simulink model "wuty_HM"  (R2019a)
settings: Solver=FixedStepAuto  StartTime=0.0  StopTime=10000  FixedStep=1  RelTol=1e-3  EnableMultiTasking=on
libraries: arduinolib x8
settings Model: SnapshotBufferSize=100  SnapshotInterval=1  ExtModeTrigDuration=2  Creator=dell  LastModifiedBy=wuty
settings SolverCC: AutoInsertRateTranBlk=on
settings DataIOCC: LimitDataPoints=on  ReturnWorkspaceOutputs=off
settings OptimizationCC: EnhancedBackFolding=on  PassReuseOutputArgsAs=Individual arguments  ZeroExternalMemoryAtStartup=off  ZeroInternalMemoryAtStartup=off  MaxStackSize=64  OptimizeBlockOrder=speed  DifferentSizesBufferReuse=on  OptimizationCustomize=off
settings DebuggingCC: ParameterTunabilityLossMsg=error  AllowSymbolicDim=off  SFUnexpectedBacktrackingDiag=warning  SFNoUnconditionalDefaultTransitionDiag=warning  SFExecutionAtInitializationDiag=none  ArithmeticOperatorsInVariantConditions=warning
settings HardwareCC: ProdBitPerInt=16  ProdBitPerPointer=16  ProdBitPerSizeT=16  ProdBitPerPtrDiffT=16  ProdLargestAtomicFloat=None  ProdWordSize=8  ProdHWDeviceType=Atmel->AVR  UseEmbeddedCoderFeatures=off
settings SFSimCC: SimUseLocalCustomCode=off  MATLABDynamicMemAlloc=off
settings RTWCC: SystemTargetFile=ert.tlc  HardwareBoard=Arduino Uno  TLCOptions=-aInlineSetEventsForThisBaseRateFcn=TLC_FALSE -aSuppressMultiTaskScheduler=TLC_FALSE -aRateBasedStepFcn=1  TemplateMakefile=ert_default_tmf  GenerateReport=on  RTWUseLocalCustomCode=off  Toolchain=Arduino AVR  BuildConfiguration=Faster Runs  IncludeHyperlinkInReport=on  LaunchReport=on  GenerateTraceInfo=on  GenerateTraceReport=on  GenerateTraceReportSl=on  GenerateTraceReportSf=on  GenerateTraceReportEml=on
settings CodeAppCC: ForceParamTrailComments=on  IgnoreCustomStorageClasses=off  OperatorAnnotations=on  SimulinkDataObjDesc=on  SFDataObjDesc=on  InsertBlockDesc=on
settings ERTTargetCC: SupportContinuousTime=on  SupportNonInlinedSFcns=on  SupportVariableSizeSignals=on  ExtModeStaticAllocSize=250
settings ConfigComp: CovMetricSettings=dw  CovHtmlReporting=on  CovSaveCumulativeToWorkspaceVar=on  CovSaveSingleToWorkspaceVar=on  CovShowResultsExplorer=off  CovExternalEMLEnable=off

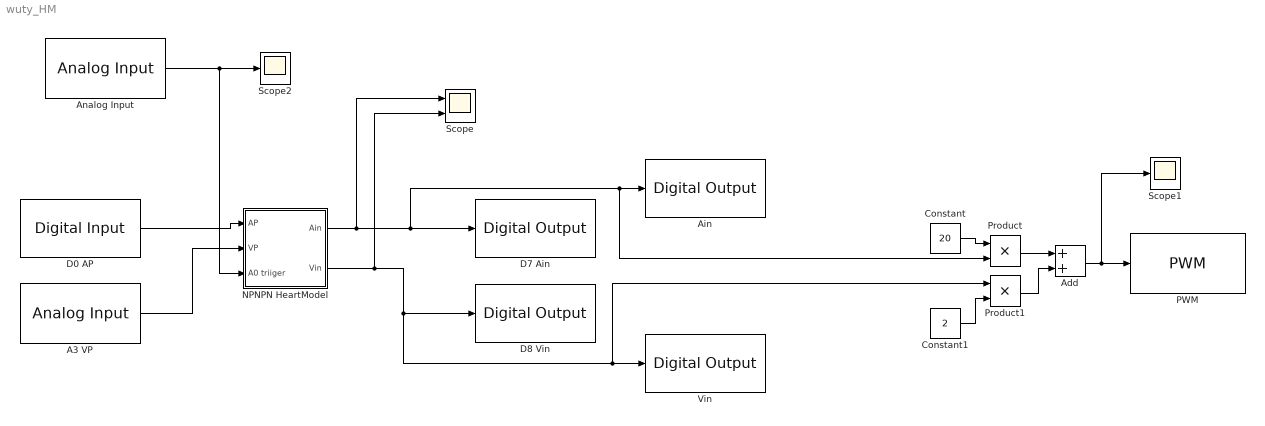
== system wuty_HM ==
  A3 VP : arduinolib/Analog Input  pinNumber=3  ReadResultsOnly=off  ConversionTriggerSource=Software  ExternalTriggerType=uint32(0)  OutputDataType=uint16  EnableConversionCompleteNotify=off  EnableOuputStatus=off  SampleTime=inf  blockPlatform=arduino
  Add : Sum
  Ain : arduinolib/Digital Output  pinNumber=13  blockPlatform=arduino
  Analog Input : arduinolib/Analog Input  pinNumber=0  ReadResultsOnly=off  ConversionTriggerSource=Software  ExternalTriggerType=uint32(0)  OutputDataType=uint16  EnableConversionCompleteNotify=off  EnableOuputStatus=off  SampleTime=inf  blockPlatform=arduino
  Constant : Constant  Value=20
  Constant1 : Constant  Value=2
  D0 AP : arduinolib/Digital Input  pinNumber=0  sampleTime=inf  blockPlatform=arduino
      settings: SourceProductName=Simulink Support Package for Arduino Hardware
  D7 Ain : arduinolib/Digital Output  pinNumber=7  blockPlatform=arduino
  D8 Vin : arduinolib/Digital Output  pinNumber=8  blockPlatform=arduino
  NPNPN HeartModel : Subsystem
  PWM : arduinolib/PWM  pinNumber=5  EnableInputFrequency=off  InitialFrequency=2000  InitialDutyCycle=0  NotificationType=None  blockPlatform=arduino
  Product : Product
  Product1 : Product
  Scope : Scope  NumInputPorts=2
  Scope1 : Scope
  Scope2 : Scope
  Vin : arduinolib/Digital Output  pinNumber=12  blockPlatform=arduino
  wires:
  NPNPN HeartModel/1(Ain) -> Scope/1, Product/2, Ain/1, D7 Ain/1
  NPNPN HeartModel/2(Vin) -> Scope/2, Product1/1, Vin/1, D8 Vin/1
  D0 AP/1 -> NPNPN HeartModel/1(AP)
  A3 VP/1 -> NPNPN HeartModel/2(VP)
  Add/1 -> Scope1/1, PWM/1
  Product/1 -> Add/1
  Constant/1 -> Product/1
  Product1/1 -> Add/2
  Constant1/1 -> Product1/2
  Analog Input/1 -> NPNPN HeartModel/3("A0 triiger "), Scope2/1

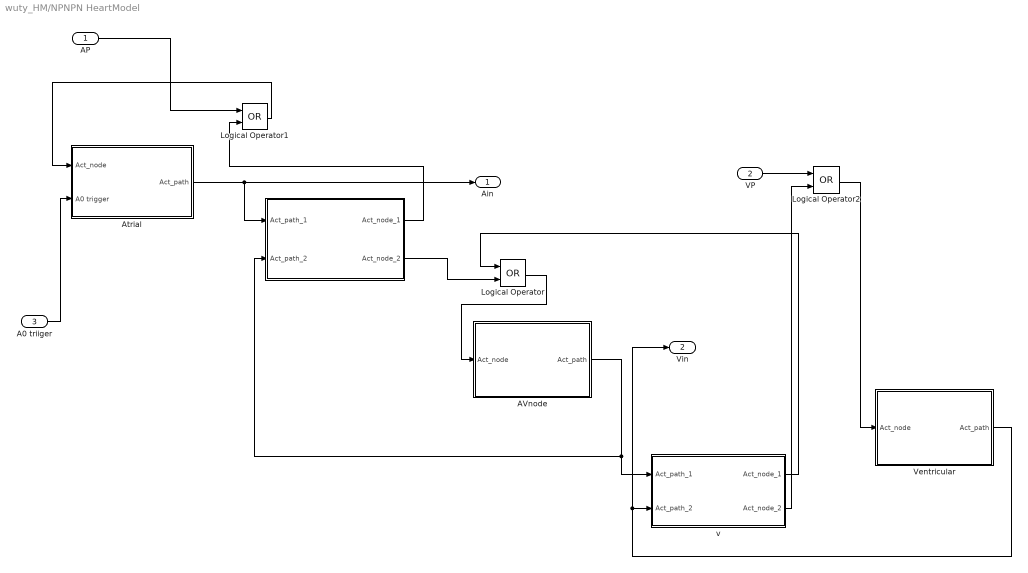
== system wuty_HM/NPNPN HeartModel ==
  AP : Inport
  VP : Inport  Port=2
  "A0 triiger " : Inport  Port=3
  " " : Subsystem  AncestorBlock=model_library/Path
  AVnode : Subsystem  AncestorBlock=model_library/Node
  Atrial : Subsystem  AncestorBlock=model_library/Node
  Logical Operator : Logic  Operator=OR  AllPortsSameDT=off  OutDataTypeStr=boolean
  Logical Operator1 : Logic  Operator=OR  AllPortsSameDT=off  OutDataTypeStr=boolean
  Logical Operator2 : Logic  Operator=OR  AllPortsSameDT=off  OutDataTypeStr=boolean
  Ventricular : Subsystem  AncestorBlock=model_library/Node
  v : Subsystem  AncestorBlock=model_library/Path
  Ain : Outport  VectorParamsAs1DForOutWhenUnconnected=on
  Vin : Outport  Port=2  VectorParamsAs1DForOutWhenUnconnected=on
  wires:
  v/1(Act_node_1) -> Logical Operator/1
  AVnode/1(Act_path) -> " "/2(Act_path_2), v/1(Act_path_1)
  Ventricular/1(Act_path) -> v/2(Act_path_2), Vin/1
  Logical Operator1/1 -> Atrial/1(Act_node)
  Logical Operator/1 -> AVnode/1(Act_node)
  " "/1(Act_node_1) -> Logical Operator1/2
  Logical Operator2/1 -> Ventricular/1(Act_node)
  " "/2(Act_node_2) -> Logical Operator/2
  v/2(Act_node_2) -> Logical Operator2/2
  Atrial/1(Act_path) -> Ain/1, " "/1(Act_path_1)
  "A0 triiger "/1 -> Atrial/2(A0 trigger)
  AP/1 -> Logical Operator1/1
  VP/1 -> Logical Operator2/1

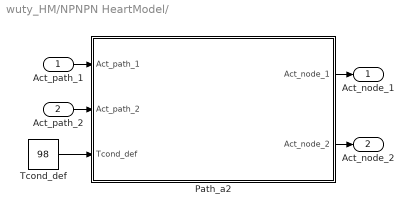
== system wuty_HM/NPNPN HeartModel/  ==
  Act_path_1 : Inport
  Act_path_2 : Inport  Port=2
  Path_a2 : Stateflow chart  TreatAsAtomicUnit=on
  Tcond_def : Constant  Value=98  OutDataTypeStr=uint16
  Act_node_1 : Outport
  Act_node_2 : Outport  Port=2
  wires:
  Tcond_def/1 -> Path_a2/3(Tcond_def)
  Path_a2/2(Act_node_2) -> Act_node_2/1
  Act_path_1/1 -> Path_a2/1(Act_path_1)
  Act_path_2/1 -> Path_a2/2(Act_path_2)
  Path_a2/1(Act_node_1) -> Act_node_1/1

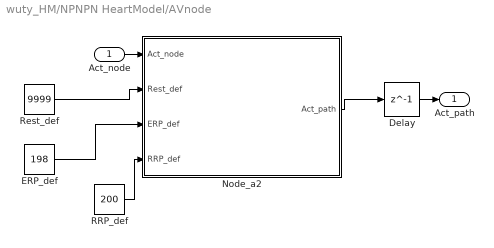
== system wuty_HM/NPNPN HeartModel/AVnode ==
  Act_node : Inport
  Delay : Delay  DelayLength=1  InitialCondition=0
  ERP_def : Constant  Value=198  OutDataTypeStr=uint16
  Node_a2 : Stateflow chart  TreatAsAtomicUnit=on
  RRP_def : Constant  Value=200  OutDataTypeStr=uint16
  Rest_def : Constant  Value=9999  OutDataTypeStr=uint16
  Act_path : Outport
  wires:
  RRP_def/1 -> Node_a2/4(RRP_def)
  Delay/1 -> Act_path/1
  ERP_def/1 -> Node_a2/3(ERP_def)
  Rest_def/1 -> Node_a2/2(Rest_def)
  Act_node/1 -> Node_a2/1(Act_node)
  Node_a2/1(Act_path) -> Delay/1

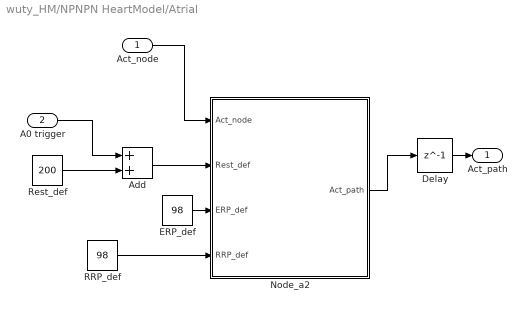
== system wuty_HM/NPNPN HeartModel/Atrial ==
  Act_node : Inport
  A0 trigger : Inport  Port=2
  Add : Sum
  Delay : Delay  DelayLength=1  InitialCondition=0
  ERP_def : Constant  Value=98  OutDataTypeStr=uint16
  Node_a2 : Stateflow chart  TreatAsAtomicUnit=on
  RRP_def : Constant  Value=98  OutDataTypeStr=uint16
  Rest_def : Constant  Value=200  OutDataTypeStr=uint16
  Act_path : Outport
  wires:
  RRP_def/1 -> Node_a2/4(RRP_def)
  Delay/1 -> Act_path/1
  ERP_def/1 -> Node_a2/3(ERP_def)
  Act_node/1 -> Node_a2/1(Act_node)
  Node_a2/1(Act_path) -> Delay/1
  Rest_def/1 -> Add/2
  A0 trigger/1 -> Add/1
  Add/1 -> Node_a2/2(Rest_def)

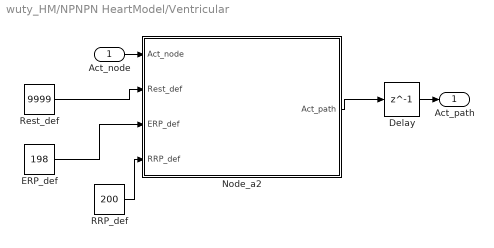
== system wuty_HM/NPNPN HeartModel/Ventricular ==
  Act_node : Inport
  Delay : Delay  DelayLength=1  InitialCondition=0
  ERP_def : Constant  Value=198  OutDataTypeStr=uint16
  Node_a2 : Stateflow chart  TreatAsAtomicUnit=on
  RRP_def : Constant  Value=200  OutDataTypeStr=uint16
  Rest_def : Constant  Value=9999  OutDataTypeStr=uint16
  Act_path : Outport
  wires:
  RRP_def/1 -> Node_a2/4(RRP_def)
  Delay/1 -> Act_path/1
  ERP_def/1 -> Node_a2/3(ERP_def)
  Rest_def/1 -> Node_a2/2(Rest_def)
  Act_node/1 -> Node_a2/1(Act_node)
  Node_a2/1(Act_path) -> Delay/1

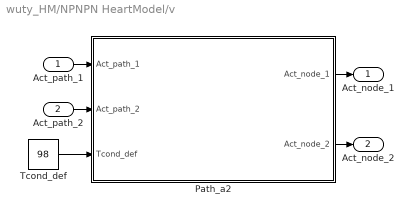
== system wuty_HM/NPNPN HeartModel/v ==
  Act_path_1 : Inport
  Act_path_2 : Inport  Port=2
  Path_a2 : Stateflow chart  TreatAsAtomicUnit=on
  Tcond_def : Constant  Value=98  OutDataTypeStr=uint16
  Act_node_1 : Outport
  Act_node_2 : Outport  Port=2
  wires:
  Tcond_def/1 -> Path_a2/3(Tcond_def)
  Path_a2/2(Act_node_2) -> Act_node_2/1
  Act_path_1/1 -> Path_a2/1(Act_path_1)
  Act_path_2/1 -> Path_a2/2(Act_path_2)
  Path_a2/1(Act_node_1) -> Act_node_1/1

== stateflow chart wuty_HM/NPNPN HeartModel/AVnode/Node_a2 ==
  state node
    settings: description=|
        | temp can be thought of a sub-mode of ERP, which only exists to make sure that act_path is high for one period.
        | 
        | In ERP, if Act_node is received, then it is ignored through that self-transition.
        | 
        | Note this doesn't model variations in cycle length because everytime it is stimulated in RRP, ERP_cur is set to ERP_def again.
    state Rest
    state RRP
    state ERP
    state temp
    (default) -> Rest : {Rest_cur=Rest_def;}
    Rest -> temp [order 3] : [Act_node==false && Rest_cur<=uint16(0)]/{Act_path=true;uptime= uint16(0);ERP_cur=ERP_def;}
    Rest -> temp [order 1] : [Act_node==true]/{Act_path=true;uptime= uint16(0);ERP_cur=ERP_def;}
    Rest -> Rest [order 2] : [Act_node==false && Rest_cur>uint16(0)]/{Rest_cur = Rest_cur - uint16(1);}
    RRP -> Rest [order 1] : [RRP_cur<=0]/{Rest_cur=Rest_def;}
    RRP -> RRP [order 2] : [Act_node==false && RRP_cur>0]/{RRP_cur=RRP_cur-uint16(1);}
    RRP -> temp [order 3] : [Act_node==true]/{Act_path=true;uptime= uint16(0);ERP_cur=ERP_def;}
    ERP -> RRP [order 1] : [ERP_cur<=uint16(0)]/{RRP_cur=RRP_def;}
    temp -> temp [order 1] : [uptime<uint16(1)]/{uptime = uptime + uint16(1);ERP_cur =ERP_cur - uint16(1);}
    temp -> ERP [order 2] : [uptime>=uint16(1)]/{Act_path=false;}
    ERP -> ERP [order 3] : [Act_node==true]
    ERP -> ERP [order 2] : {ERP_cur = ERP_cur - uint16(1);}
  data: Act_node input boolean; Act_path output boolean; Rest_cur local uint16; ERP_cur local uint16; Rest_def input uint16; ERP_def input uint16; uptime local uint16; RRP_cur local uint16; RRP_def input uint16

== stateflow chart wuty_HM/NPNPN HeartModel/v/Path_a2 ==
  state path
    state Idle
    state Ante
    state Retro
    state Wait
    (default) -> Idle
    Idle -> Ante [order 1] : [Act_path_1==true]/{Tcond_cur=Tcond_def;}
    Idle -> Retro [order 2] : [Act_path_2==true]/{Tcond_cur=Tcond_def;}
    Wait -> Idle [order 1] : [uptime>0]/{Act_node_1=false;Act_node_2=false;}
    Ante -> Ante [order 3] : [Act_path_2==false && Tcond_cur>uint16(0)]/{Tcond_cur = Tcond_cur - uint16(1);}
    Retro -> Retro [order 3] : [Act_path_1==false && Tcond_cur>uint16(0)]/{Tcond_cur = Tcond_cur - uint16(1);}
    Ante -> Wait [order 2] : [Act_path_2==true]/{uptime=uint16(0);}
    Ante -> Wait [order 1] : [Act_path_2==false && Tcond_cur<=uint16(0)]/{Act_node_2=true;uptime=uint16(0);}
    Retro -> Wait [order 2] : [Act_path_1==true]/{uptime=uint16(0);}
    Retro -> Wait [order 1] : [Act_path_1==false && Tcond_cur<=uint16(0)]/{Act_node_1=true;uptime=uint16(0);}
    Wait -> Wait [order 2] : [uptime<=uint16(0)]/{uptime = uptime + uint16(1);}
  data: Act_path_1 input boolean; Act_path_2 input boolean; Act_node_1 output boolean; Act_node_2 output boolean; Tcond_cur local uint16; Tcond_def input uint16; uptime local uint16

== stateflow chart wuty_HM/NPNPN HeartModel/Ventricular/Node_a2 ==
  state node
    settings: description=|
        | temp can be thought of a sub-mode of ERP, which only exists to make sure that act_path is high for one period.
        | 
        | In ERP, if Act_node is received, then it is ignored through that self-transition.
        | 
        | Note this doesn't model variations in cycle length because everytime it is stimulated in RRP, ERP_cur is set to ERP_def again.
    state Rest
    state RRP
    state ERP
    state temp
    (default) -> Rest : {Rest_cur=Rest_def;}
    Rest -> temp [order 3] : [Act_node==false && Rest_cur<=uint16(0)]/{Act_path=true;uptime= uint16(0);ERP_cur=ERP_def;}
    Rest -> temp [order 1] : [Act_node==true]/{Act_path=true;uptime= uint16(0);ERP_cur=ERP_def;}
    Rest -> Rest [order 2] : [Act_node==false && Rest_cur>uint16(0)]/{Rest_cur = Rest_cur - uint16(1);}
    RRP -> Rest [order 1] : [RRP_cur<=0]/{Rest_cur=Rest_def;}
    RRP -> RRP [order 2] : [Act_node==false && RRP_cur>0]/{RRP_cur=RRP_cur-uint16(1);}
    RRP -> temp [order 3] : [Act_node==true]/{Act_path=true;uptime= uint16(0);ERP_cur=ERP_def;}
    ERP -> RRP [order 1] : [ERP_cur<=uint16(0)]/{RRP_cur=RRP_def;}
    temp -> temp [order 1] : [uptime<uint16(1)]/{uptime = uptime + uint16(1);ERP_cur =ERP_cur - uint16(1);}
    temp -> ERP [order 2] : [uptime>=uint16(1)]/{Act_path=false;}
    ERP -> ERP [order 3] : [Act_node==true]
    ERP -> ERP [order 2] : {ERP_cur = ERP_cur - uint16(1);}
  data: Act_node input boolean; Act_path output boolean; Rest_cur local uint16; ERP_cur local uint16; Rest_def input uint16; ERP_def input uint16; uptime local uint16; RRP_cur local uint16; RRP_def input uint16

== stateflow chart wuty_HM/NPNPN HeartModel/Atrial/Node_a2 ==
  state node
    settings: description=|
        | temp can be thought of a sub-mode of ERP, which only exists to make sure that act_path is high for one period.
        | 
        | In ERP, if Act_node is received, then it is ignored through that self-transition.
        | 
        | Note this doesn't model variations in cycle length because everytime it is stimulated in RRP, ERP_cur is set to ERP_def again.
    state Rest
    state RRP
    state ERP
    state temp
    (default) -> Rest : {Rest_cur=Rest_def;}
    Rest -> temp [order 3] : [Act_node==false && Rest_cur<=uint16(0)]/{Act_path=true;uptime= uint16(0);ERP_cur=ERP_def;}
    Rest -> temp [order 1] : [Act_node==true]/{Act_path=true;uptime= uint16(0);ERP_cur=ERP_def;}
    Rest -> Rest [order 2] : [Act_node==false && Rest_cur>uint16(0)]/{Rest_cur = Rest_cur - uint16(1);}
    RRP -> Rest [order 1] : [RRP_cur<=0]/{Rest_cur=Rest_def;}
    RRP -> RRP [order 2] : [Act_node==false && RRP_cur>0]/{RRP_cur=RRP_cur-uint16(1);}
    RRP -> temp [order 3] : [Act_node==true]/{Act_path=true;uptime= uint16(0);ERP_cur=ERP_def;}
    ERP -> RRP [order 1] : [ERP_cur<=uint16(0)]/{RRP_cur=RRP_def;}
    temp -> temp [order 1] : [uptime<uint16(1)]/{uptime = uptime + uint16(1);ERP_cur =ERP_cur - uint16(1);}
    temp -> ERP [order 2] : [uptime>=uint16(1)]/{Act_path=false;}
    ERP -> ERP [order 3] : [Act_node==true]
    ERP -> ERP [order 2] : {ERP_cur = ERP_cur - uint16(1);}
  data: Act_node input boolean; Act_path output boolean; Rest_cur local uint16; ERP_cur local uint16; Rest_def input uint16; ERP_def input uint16; uptime local uint16; RRP_cur local uint16; RRP_def input uint16

== stateflow chart wuty_HM/NPNPN HeartModel/ /Path_a2 ==
  state path
    state Idle
    state Ante
    state Retro
    state Wait
    (default) -> Idle
    Idle -> Ante [order 1] : [Act_path_1==true]/{Tcond_cur=Tcond_def;}
    Idle -> Retro [order 2] : [Act_path_2==true]/{Tcond_cur=Tcond_def;}
    Wait -> Idle [order 1] : [uptime>0]/{Act_node_1=false;Act_node_2=false;}
    Ante -> Ante [order 3] : [Act_path_2==false && Tcond_cur>uint16(0)]/{Tcond_cur = Tcond_cur - uint16(1);}
    Retro -> Retro [order 3] : [Act_path_1==false && Tcond_cur>uint16(0)]/{Tcond_cur = Tcond_cur - uint16(1);}
    Ante -> Wait [order 2] : [Act_path_2==true]/{uptime=uint16(0);}
    Ante -> Wait [order 1] : [Act_path_2==false && Tcond_cur<=uint16(0)]/{Act_node_2=true;uptime=uint16(0);}
    Retro -> Wait [order 2] : [Act_path_1==true]/{uptime=uint16(0);}
    Retro -> Wait [order 1] : [Act_path_1==false && Tcond_cur<=uint16(0)]/{Act_node_1=true;uptime=uint16(0);}
    Wait -> Wait [order 2] : [uptime<=uint16(0)]/{uptime = uptime + uint16(1);}
  data: Act_path_1 input boolean; Act_path_2 input boolean; Act_node_1 output boolean; Act_node_2 output boolean; Tcond_cur local uint16; Tcond_def input uint16; uptime local uint16
